simulink model "H12"  (Simulink 7.3)
settings: Solver=ode45  StartTime=0.0  StopTime=2  RelTol=1e-3
settings Model: Creator=Sainquake  LastModifiedBy=Sainquake Notebook

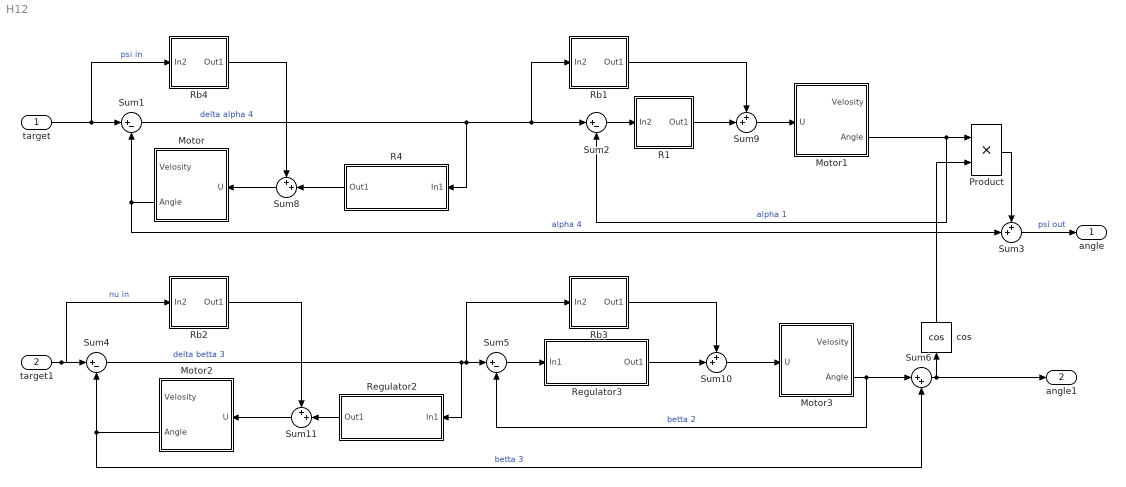
== system H12 ==
  target : Inport  OutDataType=fixdt(1, 16)  OutScaling=2^0
  target1 : Inport  Port=2  OutDataType=fixdt(1, 16)  OutScaling=2^0
  Motor : Subsystem  TreatAsAtomicUnit=on
  Motor1 : Subsystem  TreatAsAtomicUnit=on
  Motor2 : Subsystem  TreatAsAtomicUnit=on
  Motor3 : Subsystem  TreatAsAtomicUnit=on
  Product : Product  OutDataType=fixdt(1, 16)  OutScaling=2^0  RndMeth=Zero
  R1 : Subsystem
  R4 : Subsystem
  Rb1 : Subsystem
  Rb2 : Subsystem
  Rb3 : Subsystem
  Rb4 : Subsystem
  Regulator2 : Subsystem
  Regulator3 : Subsystem
  Sum{1..2,4..5} (4 alike) : Sum  Inputs=|+-  OutDataType=fixdt(1, 16)  OutScaling=2^0
  Sum{3,8..11} (5 alike) : Sum  Inputs=++|  OutDataType=fixdt(1, 16)  OutScaling=2^0
  Sum6 : Sum  Inputs=|++  OutDataType=fixdt(1, 16)  OutScaling=2^0
  cos : Trigonometry  Operator=cos
  angle : Outport  OutDataType=fixdt(1, 16)  OutScaling=2^0
  angle1 : Outport  Port=2  OutDataType=fixdt(1, 16)  OutScaling=2^0
  wires:
  R4/1(Out1) -> Sum8/2
  Motor1/2(Angle) -> Product/1, Sum2/2  "alpha 1"
  Sum2/1 -> R1/1(In2)
  Product/1 -> Sum3/1
  Sum3/1 -> angle/1  "psi out"
  Motor/2(Angle) -> Sum1/2, Sum3/2  "alpha 4"
  Regulator2/1(Out1) -> Sum11/2
  Sum4/1 -> Regulator2/1(In1), Sum5/1, Rb3/1(In2)  "delta betta 3"
  target1/1 -> Sum4/1, Rb2/1(In2)  "nu in"
  Regulator3/1(Out1) -> Sum10/2
  Motor3/2(Angle) -> Sum5/2, Sum6/1  "betta 2"
  Sum5/1 -> Regulator3/1(In1)
  Motor2/2(Angle) -> Sum4/2, Sum6/2  "betta 3"
  Sum6/1 -> cos/1, angle1/1
  cos/1 -> Product/2
  target/1 -> Sum1/1, Rb4/1(In2)  "psi in"
  Rb1/1(Out1) -> Sum9/1
  Sum1/1 -> R4/1(In1), Sum2/1, Rb1/1(In2)  "delta alpha 4"
  Rb4/1(Out1) -> Sum8/1
  R1/1(Out1) -> Sum9/2
  Sum9/1 -> Motor1/1(U)
  Sum8/1 -> Motor/1(U)
  Rb2/1(Out1) -> Sum11/1
  Sum11/1 -> Motor2/1(U)
  Sum10/1 -> Motor3/1(U)
  Rb3/1(Out1) -> Sum10/1

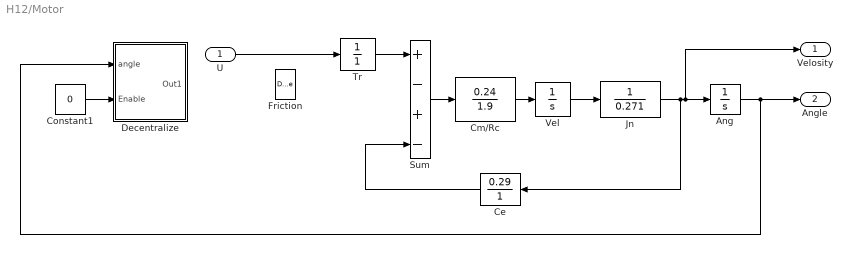
== system H12/Motor ==
  U : Inport  OutDataType=fixdt(1, 16)  OutScaling=2^0
  Ang : Integrator
  Ce : TransferFcn  Numerator=[0.29]  Denominator=[ 1]
  Cm/Rc : TransferFcn  Numerator=[0.24]  Denominator=1.9
  Constant1 : Constant  Value=0  OutDataType=fixdt(1, 16)  OutScaling=2^0
  Decentralize : Subsystem  TreatAsAtomicUnit=on
  Friction : DeadZone  LowerValue=-1.4  UpperValue=1.4  SaturateOnIntegerOverflow=on
  Jn : TransferFcn  Denominator=0.271
  Sum : Sum  Inputs=+-+-
  Tr : TransferFcn  Denominator=[ 1 ]
  Vel : Integrator
  Velosity : Outport  OutDataType=fixdt(1, 16)  OutScaling=2^0
  Angle : Outport  Port=2  OutDataType=fixdt(1, 16)  OutScaling=2^0
  wires:
  Sum/1 -> Cm/Rc/1
  Cm/Rc/1 -> Vel/1
  Ang/1 -> Decentralize/1(angle), Angle/1
  Ce/1 -> Sum/4
  Tr/1 -> Sum/1
  Constant1/1 -> Decentralize/2(Enable)
  Vel/1 -> Jn/1
  Jn/1 -> Ce/1, Ang/1, Velosity/1
  U/1 -> Tr/1

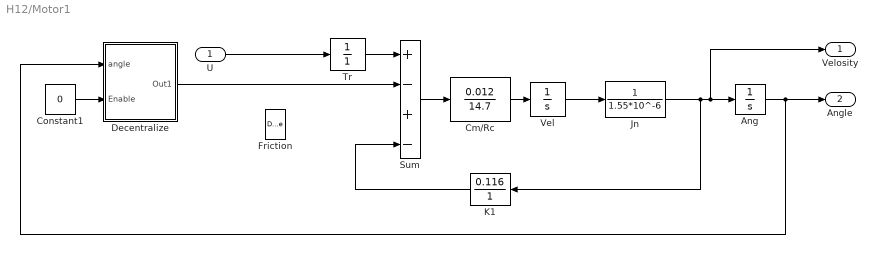
== system H12/Motor1 ==
  U : Inport  OutDataType=fixdt(1, 16)  OutScaling=2^0
  Ang : Integrator
  Cm/Rc : TransferFcn  Numerator=[0.012]  Denominator=14.7
  Constant1 : Constant  Value=0  OutDataType=fixdt(1, 16)  OutScaling=2^0
  Decentralize : Subsystem  TreatAsAtomicUnit=on
  Friction : DeadZone  LowerValue=-1.4  UpperValue=1.4  SaturateOnIntegerOverflow=on
  Jn : TransferFcn  Denominator=1.55*10^-6
  K1 : TransferFcn  Numerator=0.116  Denominator=[ 1]
  Sum : Sum  Inputs=+-+-
  Tr : TransferFcn  Numerator=1  Denominator=[ 1 ]
  Vel : Integrator
  Velosity : Outport  OutDataType=fixdt(1, 16)  OutScaling=2^0
  Angle : Outport  Port=2  OutDataType=fixdt(1, 16)  OutScaling=2^0
  wires:
  Sum/1 -> Cm/Rc/1
  Ang/1 -> Decentralize/1(angle), Angle/1
  K1/1 -> Sum/4
  Tr/1 -> Sum/1
  Decentralize/1(Out1) -> Sum/2
  Constant1/1 -> Decentralize/2(Enable)
  Jn/1 -> K1/1, Ang/1, Velosity/1
  Cm/Rc/1 -> Vel/1
  Vel/1 -> Jn/1
  U/1 -> Tr/1

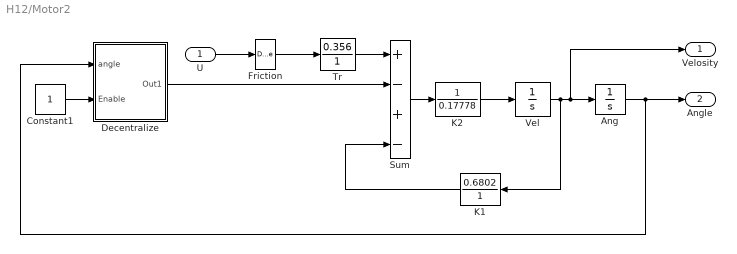
== system H12/Motor2 ==
  U : Inport  OutDataType=fixdt(1, 16)  OutScaling=2^0
  Ang : Integrator
  Constant1 : Constant  OutDataType=fixdt(1, 16)  OutScaling=2^0
  Decentralize : Subsystem  TreatAsAtomicUnit=on
  Friction : DeadZone  LowerValue=-1.4  UpperValue=1.4  SaturateOnIntegerOverflow=on
  K1 : TransferFcn  Numerator=[0.6802]  Denominator=[ 1]
  K2 : TransferFcn  Denominator=0.17778
  Sum : Sum  Inputs=+-+-
  Tr : TransferFcn  Numerator=[0.356]  Denominator=[ 1 ]
  Vel : Integrator
  Velosity : Outport  OutDataType=fixdt(1, 16)  OutScaling=2^0
  Angle : Outport  Port=2  OutDataType=fixdt(1, 16)  OutScaling=2^0
  wires:
  Sum/1 -> K2/1
  K2/1 -> Vel/1
  Ang/1 -> Decentralize/1(angle), Angle/1
  K1/1 -> Sum/4
  Tr/1 -> Sum/1
  Decentralize/1(Out1) -> Sum/2
  Friction/1 -> Tr/1
  U/1 -> Friction/1
  Constant1/1 -> Decentralize/2(Enable)
  Vel/1 -> K1/1, Ang/1, Velosity/1

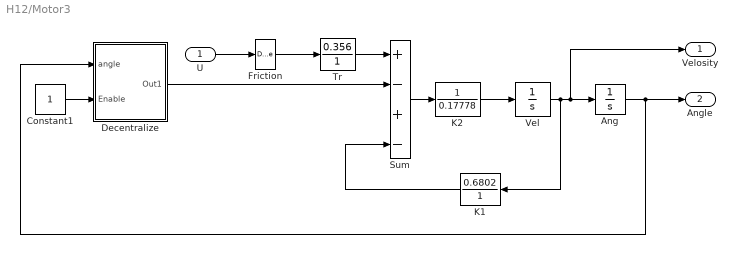
== system H12/Motor3 ==
  U : Inport  OutDataType=fixdt(1, 16)  OutScaling=2^0
  Ang : Integrator
  Constant1 : Constant  OutDataType=fixdt(1, 16)  OutScaling=2^0
  Decentralize : Subsystem  TreatAsAtomicUnit=on
  Friction : DeadZone  LowerValue=-1.4  UpperValue=1.4  SaturateOnIntegerOverflow=on
  K1 : TransferFcn  Numerator=[0.6802]  Denominator=[ 1]
  K2 : TransferFcn  Denominator=0.17778
  Sum : Sum  Inputs=+-+-
  Tr : TransferFcn  Numerator=[0.356]  Denominator=[ 1 ]
  Vel : Integrator
  Velosity : Outport  OutDataType=fixdt(1, 16)  OutScaling=2^0
  Angle : Outport  Port=2  OutDataType=fixdt(1, 16)  OutScaling=2^0
  wires:
  Sum/1 -> K2/1
  K2/1 -> Vel/1
  Ang/1 -> Decentralize/1(angle), Angle/1
  K1/1 -> Sum/4
  Tr/1 -> Sum/1
  Decentralize/1(Out1) -> Sum/2
  Friction/1 -> Tr/1
  U/1 -> Friction/1
  Constant1/1 -> Decentralize/2(Enable)
  Vel/1 -> K1/1, Ang/1, Velosity/1

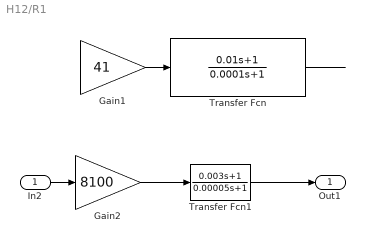
== system H12/R1 ==
  In2 : Inport  OutDataType=fixdt(1, 16)  OutScaling=2^0
  Gain1 : Gain  Gain=41  ParameterDataType=fixdt(1, 16)  ParameterScaling=2^0  OutDataType=fixdt(1, 16)  OutScaling=2^0
  Gain2 : Gain  Gain=8100  ParameterDataType=fixdt(1, 16)  ParameterScaling=2^0  OutDataType=fixdt(1, 16)  OutScaling=2^0
  Transfer Fcn : TransferFcn  Numerator=[0.01 1]  Denominator=[0.0001 1]
  Transfer Fcn1 : TransferFcn  Numerator=[0.003 1]  Denominator=[0.00005 1]
  Out1 : Outport  OutDataType=fixdt(1, 16)  OutScaling=2^0
  wires:
  Gain1/1 -> Transfer Fcn/1
  ? -> Gain1/1
  Transfer Fcn/1 -> ?
  Gain2/1 -> Transfer Fcn1/1
  In2/1 -> Gain2/1
  Transfer Fcn1/1 -> Out1/1

== system H12/R4 ==
  In1 : Inport  OutDataType=fixdt(1, 16)  OutScaling=2^0
  Gain : Gain  Gain=60  ParameterDataType=fixdt(1, 16)  ParameterScaling=2^0  OutDataType=fixdt(1, 16)  OutScaling=2^0
  Transfer Fcn : TransferFcn  Numerator=[15/60 1]  Denominator=[0.001 1]
  Out1 : Outport  OutDataType=fixdt(1, 16)  OutScaling=2^0
  wires:
  In1/1 -> Gain/1
  Gain/1 -> Transfer Fcn/1
  Transfer Fcn/1 -> Out1/1

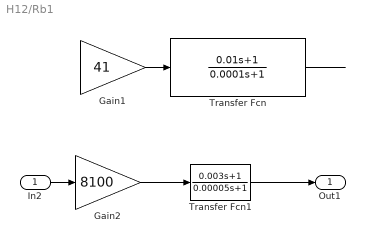
== system H12/Rb1 ==
  In2 : Inport  OutDataType=fixdt(1, 16)  OutScaling=2^0
  Gain1 : Gain  Gain=41  ParameterDataType=fixdt(1, 16)  ParameterScaling=2^0  OutDataType=fixdt(1, 16)  OutScaling=2^0
  Gain2 : Gain  Gain=8100  ParameterDataType=fixdt(1, 16)  ParameterScaling=2^0  OutDataType=fixdt(1, 16)  OutScaling=2^0
  Transfer Fcn : TransferFcn  Numerator=[0.01 1]  Denominator=[0.0001 1]
  Transfer Fcn1 : TransferFcn  Numerator=[0.003 1]  Denominator=[0.00005 1]
  Out1 : Outport  OutDataType=fixdt(1, 16)  OutScaling=2^0
  wires:
  Transfer Fcn1/1 -> Out1/1
  In2/1 -> Gain2/1
  Gain2/1 -> Transfer Fcn1/1
  Transfer Fcn/1 -> ?
  ? -> Gain1/1
  Gain1/1 -> Transfer Fcn/1

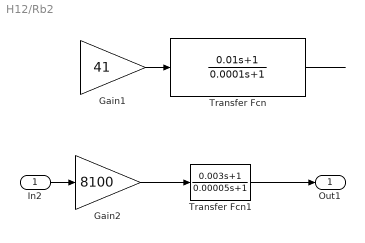
== system H12/Rb2 ==
  In2 : Inport  OutDataType=fixdt(1, 16)  OutScaling=2^0
  Gain1 : Gain  Gain=41  ParameterDataType=fixdt(1, 16)  ParameterScaling=2^0  OutDataType=fixdt(1, 16)  OutScaling=2^0
  Gain2 : Gain  Gain=8100  ParameterDataType=fixdt(1, 16)  ParameterScaling=2^0  OutDataType=fixdt(1, 16)  OutScaling=2^0
  Transfer Fcn : TransferFcn  Numerator=[0.01 1]  Denominator=[0.0001 1]
  Transfer Fcn1 : TransferFcn  Numerator=[0.003 1]  Denominator=[0.00005 1]
  Out1 : Outport  OutDataType=fixdt(1, 16)  OutScaling=2^0
  wires:
  Transfer Fcn1/1 -> Out1/1
  In2/1 -> Gain2/1
  Gain2/1 -> Transfer Fcn1/1
  Transfer Fcn/1 -> ?
  ? -> Gain1/1
  Gain1/1 -> Transfer Fcn/1

== system H12/Rb3 ==
  In2 : Inport  OutDataType=fixdt(1, 16)  OutScaling=2^0
  Gain1 : Gain  Gain=41  ParameterDataType=fixdt(1, 16)  ParameterScaling=2^0  OutDataType=fixdt(1, 16)  OutScaling=2^0
  Gain2 : Gain  Gain=8100  ParameterDataType=fixdt(1, 16)  ParameterScaling=2^0  OutDataType=fixdt(1, 16)  OutScaling=2^0
  Transfer Fcn : TransferFcn  Numerator=[0.01 1]  Denominator=[0.0001 1]
  Transfer Fcn1 : TransferFcn  Numerator=[0.003 1]  Denominator=[0.00005 1]
  Out1 : Outport  OutDataType=fixdt(1, 16)  OutScaling=2^0
  wires:
  Gain1/1 -> Transfer Fcn/1
  ? -> Gain1/1
  Transfer Fcn/1 -> ?
  Gain2/1 -> Transfer Fcn1/1
  In2/1 -> Gain2/1
  Transfer Fcn1/1 -> Out1/1

== system H12/Rb4 ==
  In2 : Inport  OutDataType=fixdt(1, 16)  OutScaling=2^0
  Gain1 : Gain  Gain=41  ParameterDataType=fixdt(1, 16)  ParameterScaling=2^0  OutDataType=fixdt(1, 16)  OutScaling=2^0
  Gain2 : Gain  Gain=8100  ParameterDataType=fixdt(1, 16)  ParameterScaling=2^0  OutDataType=fixdt(1, 16)  OutScaling=2^0
  Transfer Fcn : TransferFcn  Numerator=[0.01 1]  Denominator=[0.0001 1]
  Transfer Fcn1 : TransferFcn  Numerator=[0.003 1]  Denominator=[0.00005 1]
  Out1 : Outport  OutDataType=fixdt(1, 16)  OutScaling=2^0
  wires:
  Gain1/1 -> Transfer Fcn/1
  ? -> Gain1/1
  Transfer Fcn/1 -> ?
  Gain2/1 -> Transfer Fcn1/1
  In2/1 -> Gain2/1
  Transfer Fcn1/1 -> Out1/1

== system H12/Regulator2 ==
  In1 : Inport  OutDataType=fixdt(1, 16)  OutScaling=2^0
  Out1 : Outport  OutDataType=fixdt(1, 16)  OutScaling=2^0
  wires:
  In1/1 -> Out1/1

== system H12/Regulator3 ==
  In1 : Inport  OutDataType=fixdt(1, 16)  OutScaling=2^0
  Out1 : Outport  OutDataType=fixdt(1, 16)  OutScaling=2^0
  wires:
  In1/1 -> Out1/1

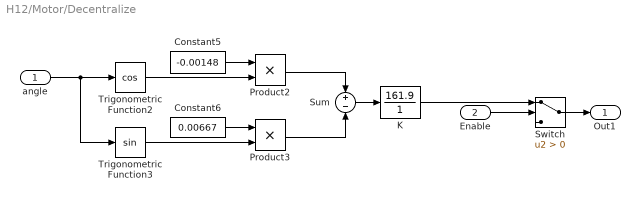
== system H12/Motor/Decentralize ==
  angle : Inport  OutDataType=fixdt(1, 16)  OutScaling=2^0
  Enable : Inport  Port=2  OutDataType=fixdt(1, 16)  OutScaling=2^0
  Constant5 : Constant  Value=-0.00148
  Constant6 : Constant  Value=0.00667
  K : TransferFcn  Numerator=[161.9]  Denominator=[ 1 ]
  Product2 : Product  RndMeth=Zero
  Product3 : Product  RndMeth=Zero
  Sum : Sum  Inputs=+|-  OutDataType=fixdt(1, 16)  OutScaling=2^0
  Switch : Switch  Criteria=u2 > Threshold  OutDataType=fixdt(1, 16)  OutScaling=2^0
  Trigonometric Function2 : Trigonometry  Operator=cos
  Trigonometric Function3 : Trigonometry
  Out1 : Outport  OutDataType=fixdt(1, 16)  OutScaling=2^0
  wires:
  Constant5/1 -> Product2/1
  Trigonometric Function2/1 -> Product2/2
  Constant6/1 -> Product3/1
  Trigonometric Function3/1 -> Product3/2
  Product3/1 -> Sum/2
  Product2/1 -> Sum/1
  Sum/1 -> K/1
  K/1 -> Switch/1
  angle/1 -> Trigonometric Function2/1, Trigonometric Function3/1
  Enable/1 -> Switch/2
  Switch/1 -> Out1/1

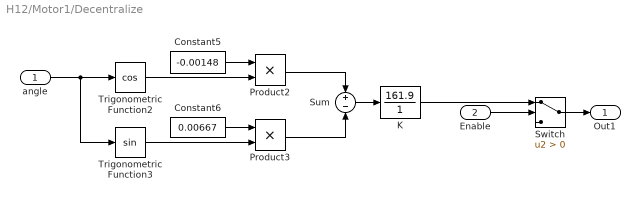
== system H12/Motor1/Decentralize ==
  angle : Inport  OutDataType=fixdt(1, 16)  OutScaling=2^0
  Enable : Inport  Port=2  OutDataType=fixdt(1, 16)  OutScaling=2^0
  Constant5 : Constant  Value=-0.00148
  Constant6 : Constant  Value=0.00667
  K : TransferFcn  Numerator=[161.9]  Denominator=[ 1 ]
  Product2 : Product  RndMeth=Zero
  Product3 : Product  RndMeth=Zero
  Sum : Sum  Inputs=+|-  OutDataType=fixdt(1, 16)  OutScaling=2^0
  Switch : Switch  Criteria=u2 > Threshold  OutDataType=fixdt(1, 16)  OutScaling=2^0
  Trigonometric Function2 : Trigonometry  Operator=cos
  Trigonometric Function3 : Trigonometry
  Out1 : Outport  OutDataType=fixdt(1, 16)  OutScaling=2^0
  wires:
  Constant5/1 -> Product2/1
  Trigonometric Function2/1 -> Product2/2
  Constant6/1 -> Product3/1
  Trigonometric Function3/1 -> Product3/2
  Product3/1 -> Sum/2
  Product2/1 -> Sum/1
  Sum/1 -> K/1
  K/1 -> Switch/1
  angle/1 -> Trigonometric Function2/1, Trigonometric Function3/1
  Enable/1 -> Switch/2
  Switch/1 -> Out1/1

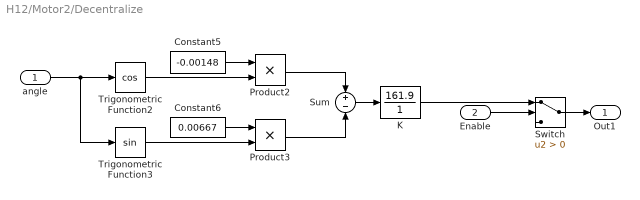
== system H12/Motor2/Decentralize ==
  angle : Inport  OutDataType=fixdt(1, 16)  OutScaling=2^0
  Enable : Inport  Port=2  OutDataType=fixdt(1, 16)  OutScaling=2^0
  Constant5 : Constant  Value=-0.00148
  Constant6 : Constant  Value=0.00667
  K : TransferFcn  Numerator=[161.9]  Denominator=[ 1 ]
  Product2 : Product  RndMeth=Zero
  Product3 : Product  RndMeth=Zero
  Sum : Sum  Inputs=+|-  OutDataType=fixdt(1, 16)  OutScaling=2^0
  Switch : Switch  Criteria=u2 > Threshold  OutDataType=fixdt(1, 16)  OutScaling=2^0
  Trigonometric Function2 : Trigonometry  Operator=cos
  Trigonometric Function3 : Trigonometry
  Out1 : Outport  OutDataType=fixdt(1, 16)  OutScaling=2^0
  wires:
  Constant5/1 -> Product2/1
  Trigonometric Function2/1 -> Product2/2
  Constant6/1 -> Product3/1
  Trigonometric Function3/1 -> Product3/2
  Product3/1 -> Sum/2
  Product2/1 -> Sum/1
  Sum/1 -> K/1
  K/1 -> Switch/1
  angle/1 -> Trigonometric Function2/1, Trigonometric Function3/1
  Enable/1 -> Switch/2
  Switch/1 -> Out1/1

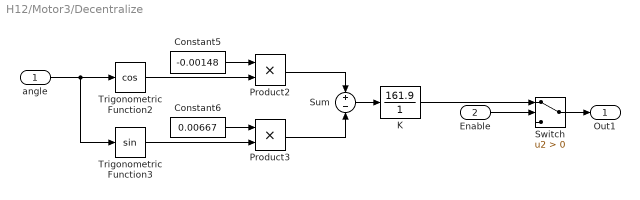
== system H12/Motor3/Decentralize ==
  angle : Inport  OutDataType=fixdt(1, 16)  OutScaling=2^0
  Enable : Inport  Port=2  OutDataType=fixdt(1, 16)  OutScaling=2^0
  Constant5 : Constant  Value=-0.00148
  Constant6 : Constant  Value=0.00667
  K : TransferFcn  Numerator=[161.9]  Denominator=[ 1 ]
  Product2 : Product  RndMeth=Zero
  Product3 : Product  RndMeth=Zero
  Sum : Sum  Inputs=+|-  OutDataType=fixdt(1, 16)  OutScaling=2^0
  Switch : Switch  Criteria=u2 > Threshold  OutDataType=fixdt(1, 16)  OutScaling=2^0
  Trigonometric Function2 : Trigonometry  Operator=cos
  Trigonometric Function3 : Trigonometry
  Out1 : Outport  OutDataType=fixdt(1, 16)  OutScaling=2^0
  wires:
  Constant5/1 -> Product2/1
  Trigonometric Function2/1 -> Product2/2
  Constant6/1 -> Product3/1
  Trigonometric Function3/1 -> Product3/2
  Product3/1 -> Sum/2
  Product2/1 -> Sum/1
  Sum/1 -> K/1
  K/1 -> Switch/1
  angle/1 -> Trigonometric Function2/1, Trigonometric Function3/1
  Enable/1 -> Switch/2
  Switch/1 -> Out1/1
